simulink model "ch5example6"  (Simulink 5.0)
settings: Solver=ode5  StartTime=0.0  StopTime=10.0  FixedStep=1/1e6  RelTol=1e-3
libraries: dsparch4 x5, simulink x2, dspswit3 x1, commcontsrc2 x1
settings Model: LastModifiedBy=lenovo

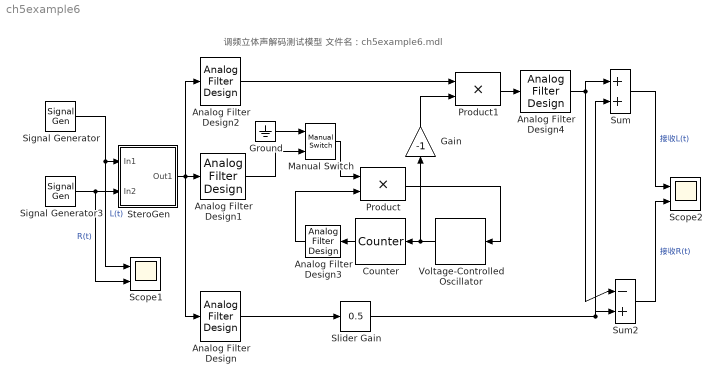
== system ch5example6 ==
  note: 调频立体声解码测试模型
      | 文件名：ch5example6.mdl
  Analog Filter Design : dsparch4/Analog Filter Design  method=Butterworth  filttype=Lowpass  N=8  Wlo=2*pi*15e3  Whi=80  Rp=2  Rs=40
  Analog Filter Design1 : dsparch4/Analog Filter Design  method=Butterworth  filttype=Bandpass  N=2  Wlo=2*pi*16e3  Whi=2*pi*20e3  Rp=2  Rs=40
  Analog Filter Design2 : dsparch4/Analog Filter Design  method=Butterworth  filttype=Bandpass  N=2  Wlo=2*pi*23e3  Whi=2*pi*53e3  Rp=2  Rs=40
  Analog Filter Design3 : dsparch4/Analog Filter Design  Orientation=left  method=Butterworth  filttype=Bandpass  N=2  Wlo=2*pi*17e3  Whi=2*pi*20e3  Rp=2  Rs=40
  Analog Filter Design4 : dsparch4/Analog Filter Design  method=Butterworth  filttype=Lowpass  N=8  Wlo=2*pi*15e3  Whi=80  Rp=2  Rs=40
  Counter : dspswit3/Counter  Orientation=left  Direction=Up  CountEvent=Rising edge  CounterSize=User defined  MaxCount=1  InitialCount=0  Output=Count  HitValue=1  ResetInput=off  SamplesPerFrame=1  Ts=1  CntDtype=Double  HitDtype=Logical
  Gain : Gain  Orientation=up  Gain=-1  SaturateOnIntegerOverflow=on
  Ground : Ground
  Manual Switch : simulink/Signal Routing/Manual Switch  sw=0  action=0
  Product : Product  SaturateOnIntegerOverflow=on
  Product1 : Product  SaturateOnIntegerOverflow=on
  Scope1 : Scope  NumInputPorts=2
      settings: TimeRange=0.002  YMin=-5~-4  YMax=5~3
  Scope2 : Scope  NumInputPorts=2
      settings: TimeRange=0.002  YMin=-6~-4  YMax=5~3
  Signal Generator : SignalGenerator  Amplitude=5  Frequency=1000
  Signal Generator3 : SignalGenerator  Amplitude=2  Frequency=2000
  Slider Gain : simulink/Math Operations/Slider Gain  low=0  gain=0.5  high=2
  SteroGen : Subsystem
  Sum : Sum  Inputs=|++  SaturateOnIntegerOverflow=on
  Sum2 : Sum  Inputs=|-+  SaturateOnIntegerOverflow=on
  Voltage-Controlled Oscillator : commcontsrc2/Voltage-Controlled Oscillator  Orientation=left  Ac=1  Fc=38e3+20  Kc=500  Ph=0
  wires:
  Signal Generator/1 -> SteroGen/1(In1), Scope1/1  "L(t)"
  Signal Generator3/1 -> SteroGen/2(In2), Scope1/2  "R(t)"
  SteroGen/1(Out1) -> Analog Filter Design1/1, Analog Filter Design2/1, Analog Filter Design/1
  Counter/1 -> Analog Filter Design3/1
  Product/1 -> Voltage-Controlled Oscillator/1
  Voltage-Controlled Oscillator/1 -> Counter/1, Gain/1
  Analog Filter Design3/1 -> Product/2
  Analog Filter Design2/1 -> Product1/1
  Product1/1 -> Analog Filter Design4/1
  Analog Filter Design/1 -> Slider Gain/1
  Analog Filter Design4/1 -> Sum/1, Sum2/1
  Slider Gain/1 -> Sum/2, Sum2/2
  Sum/1 -> Scope2/1  "接收L(t)"
  Sum2/1 -> Scope2/2  "接收R(t)"
  Gain/1 -> Product1/2
  Analog Filter Design1/1 -> Manual Switch/2
  Manual Switch/1 -> Product/1
  Ground/1 -> Manual Switch/1

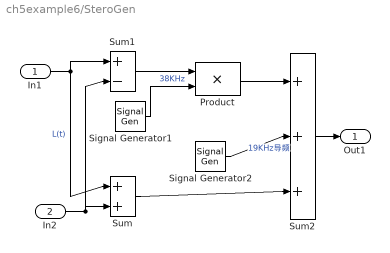
== system ch5example6/SteroGen ==
  In1 : Inport
  In2 : Inport  Port=2
  Product : Product  SaturateOnIntegerOverflow=on
  Signal Generator1 : SignalGenerator  Frequency=38e3
  Signal Generator2 : SignalGenerator  Frequency=19e3
  Sum : Sum  Inputs=|++  SaturateOnIntegerOverflow=on
  Sum1 : Sum  Inputs=|+-  SaturateOnIntegerOverflow=on
  Sum2 : Sum  Inputs=|+++  SaturateOnIntegerOverflow=on
  Out1 : Outport
  wires:
  In1/1 -> Sum1/1, Sum/1  "L(t)"
  In2/1 -> Sum1/2, Sum/2
  Sum1/1 -> Product/1
  Signal Generator1/1 -> Product/2  "38KHz"
  Product/1 -> Sum2/1
  Signal Generator2/1 -> Sum2/2  "19KHz导频"
  Sum/1 -> Sum2/3
  Sum2/1 -> Out1/1
